simulink library "lib_decmp_Calib_pirelle_presSnr_x8"  (R2020a)
settings: Solver=VariableStepAuto  StartTime=0.0  StopTime=10.0  RelTol=1e-3
settings Model: Creator=Administrator  LastModifiedBy=Administrator

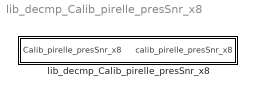
== system lib_decmp_Calib_pirelle_presSnr_x8 ==
  lib_decmp_Calib_pirelle_presSnr_x8 : Subsystem

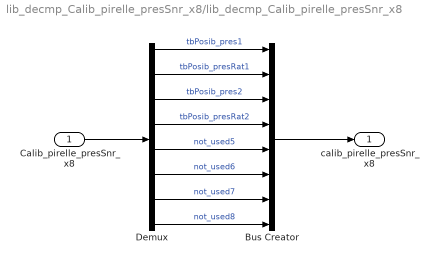
== system lib_decmp_Calib_pirelle_presSnr_x8/lib_decmp_Calib_pirelle_presSnr_x8 ==
  Calib_pirelle_presSnr_x8 : Inport  OutDataTypeStr=single  PortDimensions=8
  Bus Creator : BusCreator  Inputs=8
  Demux : Demux  Outputs=8
  calib_pirelle_presSnr_x8 : Outport  PortDimensions=8
  wires:
  Calib_pirelle_presSnr_x8/1 -> Demux/1
  Demux/1 -> Bus Creator/1  "tbPosib_pres1"
  Demux/2 -> Bus Creator/2  "tbPosib_presRat1"
  Demux/3 -> Bus Creator/3  "tbPosib_pres2"
  Demux/4 -> Bus Creator/4  "tbPosib_presRat2"
  Bus Creator/1 -> calib_pirelle_presSnr_x8/1
  Demux/5 -> Bus Creator/5  "not_used5"
  Demux/6 -> Bus Creator/6  "not_used6"
  Demux/7 -> Bus Creator/7  "not_used7"
  Demux/8 -> Bus Creator/8  "not_used8"
